simulink model "Ericc_correction"  (R2015b)
settings: Solver=ode45  StartTime=0.0  StopTime=1  MaxStep=0.01  RelTol=1e-3
values from neighbouring files (symbols this model uses):
  Cfsec = 1    [para.m]
  DAC = 1    [para.m]
  f = 8.06e-5    (= 8.06e-05)    [para.m]
  Jeq = 2.9e-5    (= 2.9e-05)    [para.m]
  Kc = 0.042    [para.m]
  Kd = 0    [para.m]
  Ki = 0    [para.m]
  Kp = 1000    [para.m]
undefined symbols (not defined in the file or in its folder): Cext
settings Model: Creator=antomart  LastModifiedBy=David
settings DataIOCC: LimitDataPoints=off  SaveFormat=StructureWithTime
settings HardwareCC: ProdWordSize=32  ProdHWDeviceType=Specified
settings ModelReferenceCC: PropagateSignalLabelsOutOfModel=on
settings GRTTargetCC: GeneratePreprocessorConditionals=Disable all

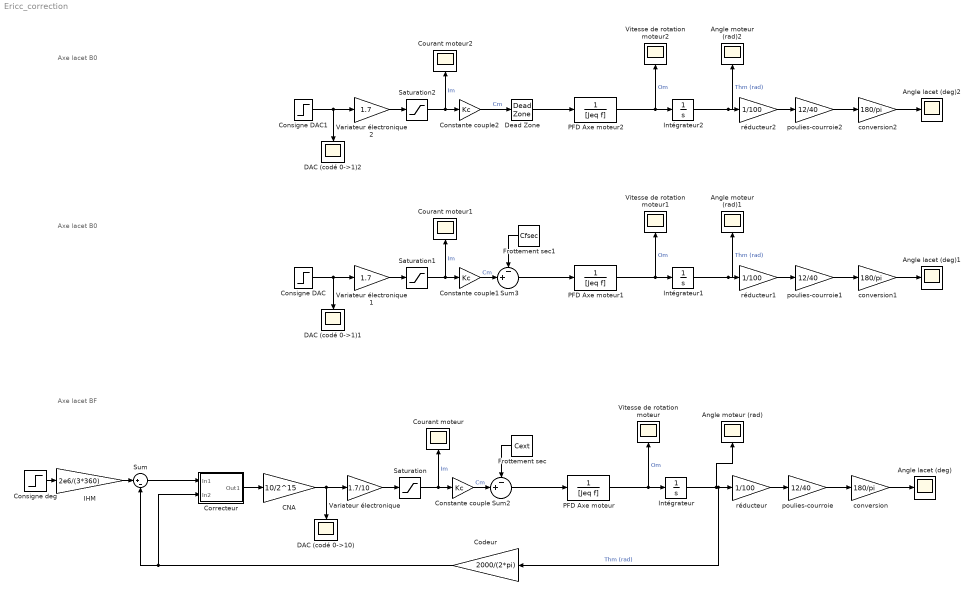
== system Ericc_correction ==
  note: Axe lacet BF
  note: Axe lacet B0
  note: Axe lacet B0
  Angle moteur (rad) : Scope
  Angle moteur (rad)1 : Scope
  Angle moteur (rad)2 : Scope
  Angle lacet (deg) : Scope
  Angle lacet (deg)1 : Scope
  Angle lacet (deg)2 : Scope
  CNA : Gain  Gain=10/2^15
  Codeur : Gain  Gain=2000/(2*pi)
  Consigne DAC : Step  Time=0  After=DAC  SampleTime=0
  Consigne DAC1 : Step  Time=0  After=DAC  SampleTime=0
  Consigne deg : Step  Time=0  After=30  SampleTime=0
  Constante couple : Gain  Gain=Kc
  Constante couple1 : Gain  Gain=Kc
  Constante couple2 : Gain  Gain=Kc
  Correcteur : Subsystem
  Courant moteur : Scope
  Courant moteur1 : Scope
  Courant moteur2 : Scope
  DAC (codé 0->1)1 : Scope
  DAC (codé 0->1)2 : Scope
  DAC (codé 0->10) : Scope
  Dead Zone : DeadZone  LowerValue=-Cfsec  UpperValue=Cfsec  SaturateOnIntegerOverflow=on
  Frottement sec : Constant  Value=Cext
  Frottement sec1 : Constant  Value=Cfsec
  IHM : Gain  Gain=2e6/(3*360)
  Intégrateur : Integrator
  Intégrateur1 : Integrator
  Intégrateur2 : Integrator
  PFD Axe moteur : TransferFcn  Denominator=[Jeq f]
  PFD Axe moteur1 : TransferFcn  Denominator=[Jeq f]
  PFD Axe moteur2 : TransferFcn  Denominator=[Jeq f]
  Saturation : Saturate  UpperLimit=1.7  LowerLimit=-1.7
  Saturation1 : Saturate  UpperLimit=1.7  LowerLimit=-1.7
  Saturation2 : Saturate  UpperLimit=1.7  LowerLimit=-1.7
  Sum : Sum  Inputs=|+-
  Sum2 : Sum  Inputs=-+|
  Sum3 : Sum  Inputs=-+|
  Variateur électronique : Gain  Gain=1.7/10
  Variateur électronique1 : Gain  Gain=1.7
  Variateur électronique2 : Gain  Gain=1.7
  Vitesse de rotation moteur : Scope
  Vitesse de rotation moteur1 : Scope
  Vitesse de rotation moteur2 : Scope
  conversion : Gain  Gain=180/pi
  conversion1 : Gain  Gain=180/pi
  conversion2 : Gain  Gain=180/pi
  poulies-courroie : Gain  Gain=12/40
  poulies-courroie1 : Gain  Gain=12/40
  poulies-courroie2 : Gain  Gain=12/40
  réducteur : Gain  Gain=1/100
  réducteur1 : Gain  Gain=1/100
  réducteur2 : Gain  Gain=1/100
  wires:
  PFD Axe moteur/1 -> Intégrateur/1, Vitesse de rotation moteur/1  "Om"
  Intégrateur/1 -> Codeur/1, réducteur/1, Angle moteur (rad)/1  "Thm (rad)"
  réducteur/1 -> poulies-courroie/1
  Sum/1 -> Correcteur/1(In1)
  Correcteur/1(Out1) -> CNA/1
  Consigne deg/1 -> IHM/1
  Codeur/1 -> Correcteur/2(In2), Sum/2
  IHM/1 -> Sum/1
  conversion/1 -> Angle lacet (deg)/1
  Sum2/1 -> PFD Axe moteur/1
  Frottement sec/1 -> Sum2/1
  Constante couple/1 -> Sum2/2  "Cm"
  Variateur électronique/1 -> Saturation/1
  CNA/1 -> Variateur électronique/1, DAC (codé 0->10)/1
  poulies-courroie/1 -> conversion/1
  Saturation/1 -> Constante couple/1, Courant moteur/1  "Im"
  PFD Axe moteur1/1 -> Intégrateur1/1, Vitesse de rotation moteur1/1  "Om"
  Intégrateur1/1 -> réducteur1/1, Angle moteur (rad)1/1  "Thm (rad)"
  réducteur1/1 -> poulies-courroie1/1
  conversion1/1 -> Angle lacet (deg)1/1
  Sum3/1 -> PFD Axe moteur1/1
  Frottement sec1/1 -> Sum3/1
  Constante couple1/1 -> Sum3/2  "Cm"
  Variateur électronique1/1 -> Saturation1/1
  Consigne DAC/1 -> Variateur électronique1/1, DAC (codé 0->1)1/1
  poulies-courroie1/1 -> conversion1/1
  Saturation1/1 -> Constante couple1/1, Courant moteur1/1  "Im"
  PFD Axe moteur2/1 -> Intégrateur2/1, Vitesse de rotation moteur2/1  "Om"
  Intégrateur2/1 -> réducteur2/1, Angle moteur (rad)2/1  "Thm (rad)"
  réducteur2/1 -> poulies-courroie2/1
  conversion2/1 -> Angle lacet (deg)2/1
  Dead Zone/1 -> PFD Axe moteur2/1
  Constante couple2/1 -> Dead Zone/1  "Cm"
  Variateur électronique2/1 -> Saturation2/1
  Consigne DAC1/1 -> Variateur électronique2/1, DAC (codé 0->1)2/1
  poulies-courroie2/1 -> conversion2/1
  Saturation2/1 -> Constante couple2/1, Courant moteur2/1  "Im"

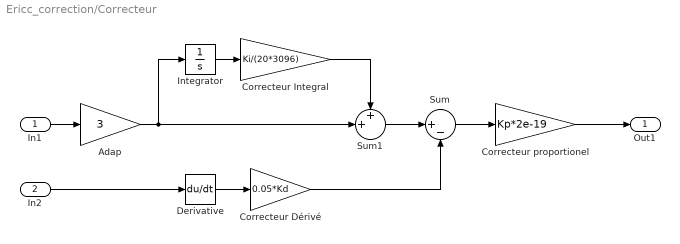
== system Ericc_correction/Correcteur ==
  In1 : Inport
  In2 : Inport  Port=2
  Adap : Gain  Gain=3
  Correcteur Dérivé : Gain  Gain=0.05*Kd
  Correcteur Integral : Gain  Gain=Ki/(20*3096)
  Correcteur proportionel : Gain  Gain=Kp*2e-19
  Derivative : Derivative
  Integrator : Integrator
  Sum : Sum  Inputs=|+-
  Sum1 : Sum  Inputs=++|
  Out1 : Outport
  wires:
  In1/1 -> Adap/1
  Integrator/1 -> Correcteur Integral/1
  Derivative/1 -> Correcteur Dérivé/1
  Correcteur Dérivé/1 -> Sum/2
  Sum/1 -> Correcteur proportionel/1
  Adap/1 -> Sum1/2, Integrator/1
  Correcteur proportionel/1 -> Out1/1
  In2/1 -> Derivative/1
  Sum1/1 -> Sum/1
  Correcteur Integral/1 -> Sum1/1
